simulink model "mavsim_chap6_week1"  (R2020b)
settings: Solver=ode4  StartTime=0.0  StopTime=tsim  FixedStep=P.Ts  RelTol=1e-3  EnableMultiTasking=on
InitFcn:
  | param_chap6
values from neighbouring files (symbols this model uses):
  aileron_c_sat = delta_a_max    (= 0.785398163397)    [runSim.m]
  closedLoopEnable = 1    [runSim.m]
  phi_c_sat = 45*pi/180    (= 0.785398163397)    [runSim.m]
undefined symbols (not defined in the file or in its folder): calc_chi, forces_moments, get_p, get_phi, P
libraries: simulink x3, pid_lib x2
settings Model: Creator=beard  LastModifiedBy=alanf
settings DataIOCC: LimitDataPoints=on  SaveFormat=Array  ReturnWorkspaceOutputs=off
settings OptimizationCC: ExpressionDepthLimit=2147483647  InitFltsAndDblsToZero=on  LifeSpan=inf
settings DebuggingCC: UnderspecifiedInitializationDetection=Classic  MergeDetectMultiDrivingBlocksExec=none  SolverPrmCheckMsg=warning  FcnCallInpInsideContextMsg=warning  StateNameClashWarn=warning  SFUnexpectedBacktrackingDiag=warning  SFNoUnconditionalDefaultTransitionDiag=warning  SFExecutionAtInitializationDiag=none  ArithmeticOperatorsInVariantConditions=warning
settings HardwareCC: ProdBitPerPointer=32  ProdBitPerSizeT=32  ProdBitPerPtrDiffT=32  ProdLargestAtomicFloat=None  ProdIntDivRoundTo=Undefined  ProdEndianess=Unspecified  ProdWordSize=32  ProdHWDeviceType=32-bit Generic
settings ModelReferenceCC: PropagateSignalLabelsOutOfModel=off
settings SFSimCC: SimUseLocalCustomCode=off  CustomCodeUndefinedFunction=UseInterfaceOnly
settings RTWCC: RTWUseLocalCustomCode=off
settings CodeAppCC: StateflowObjectComments=on
settings GRTTargetCC: TargetLangStandard=C89/C90 (ANSI)  CombineOutputUpdateFcns=off  GRTInterface=on
settings ConfigComp: CovMetricSettings=dw  CovSaveCumulativeToWorkspaceVar=on  CovSaveSingleToWorkspaceVar=on  CovExternalEMLEnable=off  CovSFcnEnable=off

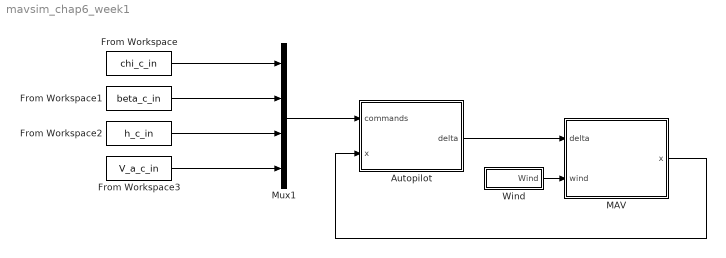
== system mavsim_chap6_week1 ==
  Autopilot : Subsystem
      mask Display: image(imread('kestrel.jpg'))
  From Workspace : FromWorkspace  VariableName=chi_c_in
  From Workspace1 : FromWorkspace  VariableName=beta_c_in
  From Workspace2 : FromWorkspace  VariableName=h_c_in
  From Workspace3 : FromWorkspace  VariableName=V_a_c_in
  MAV : Subsystem
      mask Display: image(imread('batcam.png'))
  Mux1 : Mux
  Wind : Subsystem
  wires:
  Wind/1(Wind) -> MAV/2(wind)
  MAV/1(x) -> Autopilot/2(x)
  Autopilot/1(delta) -> MAV/1(delta)
  Mux1/1 -> Autopilot/1(commands)
  From Workspace/1 -> Mux1/1
  From Workspace1/1 -> Mux1/2
  From Workspace2/1 -> Mux1/3
  From Workspace3/1 -> Mux1/4

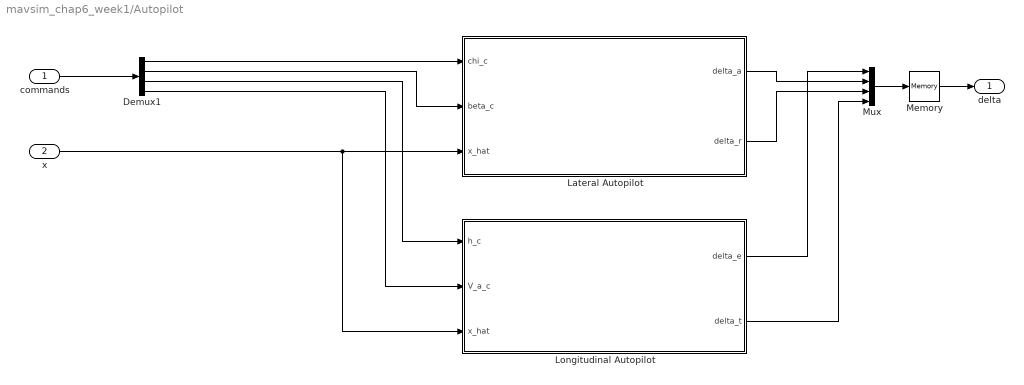
== system mavsim_chap6_week1/Autopilot ==
  commands : Inport
  x : Inport  Port=2
  Demux1 : Demux
  Lateral Autopilot : Subsystem
  Longitudinal Autopilot : Subsystem
  Memory : Memory  InitialCondition=P.u_trim  InheritSampleTime=on
  Mux : Mux
  delta : Outport  VectorParamsAs1DForOutWhenUnconnected=off
  wires:
  x/1 -> Longitudinal Autopilot/3(x_hat), Lateral Autopilot/3(x_hat)
  commands/1 -> Demux1/1
  Demux1/1 -> Lateral Autopilot/1(chi_c)
  Demux1/2 -> Lateral Autopilot/2(beta_c)
  Demux1/3 -> Longitudinal Autopilot/1(h_c)
  Demux1/4 -> Longitudinal Autopilot/2(V_a_c)
  Mux/1 -> Memory/1
  Memory/1 -> delta/1
  Longitudinal Autopilot/1(delta_e) -> Mux/1
  Lateral Autopilot/1(delta_a) -> Mux/2
  Lateral Autopilot/2(delta_r) -> Mux/3
  Longitudinal Autopilot/2(delta_t) -> Mux/4

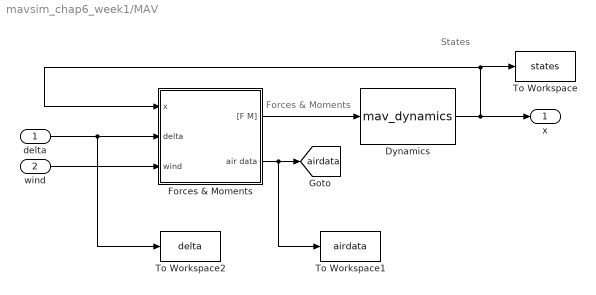
== system mavsim_chap6_week1/MAV ==
  note: Forces & Moments
  note: States
  delta : Inport
  wind : Inport  Port=2
  Dynamics : S-Function  FunctionName=mav_dynamics  Parameters=P  SFunctionDeploymentMode=off  EnableBusSupport=off
  Forces & Moments : Subsystem
  To Workspace : ToWorkspace  VariableName=states  SaveFormat=Timeseries  SampleTime=-1
  To Workspace1 : ToWorkspace  VariableName=airdata  SaveFormat=Timeseries  SampleTime=-1
  To Workspace2 : ToWorkspace  VariableName=delta  SaveFormat=Timeseries  SampleTime=-1
  x : Outport  VectorParamsAs1DForOutWhenUnconnected=off
  tag scope: airdata=global
  wires:
  Dynamics/1 -> Forces & Moments/1(x), To Workspace/1, x/1
  Forces & Moments/1("[F M]") -> Dynamics/1
  Forces & Moments/2(air data) -> To Workspace1/1, [airdata]
  delta/1 -> To Workspace2/1, Forces & Moments/2(delta)
  wind/1 -> Forces & Moments/3(wind)

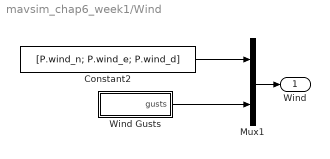
== system mavsim_chap6_week1/Wind ==
  Constant2 : Constant  Value=[P.wind_n; P.wind_e; P.wind_d]
  Mux1 : Mux  Inputs=2
  Wind Gusts : Subsystem
  Wind : Outport  VectorParamsAs1DForOutWhenUnconnected=off
  wires:
  Constant2/1 -> Mux1/1
  Mux1/1 -> Wind/1
  Wind Gusts/1(gusts) -> Mux1/2

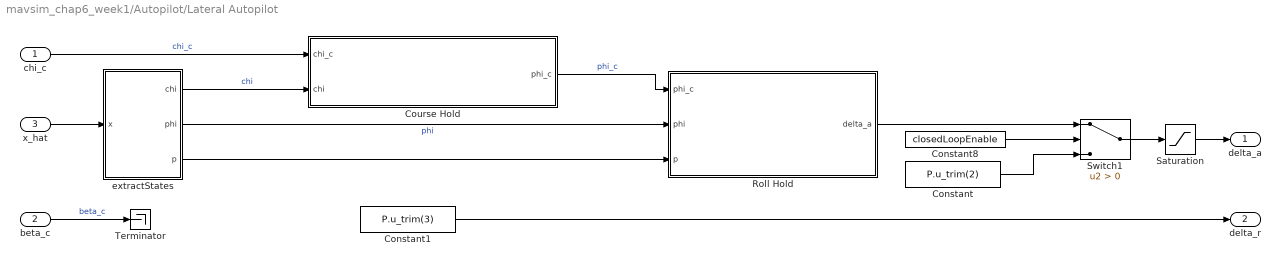
== system mavsim_chap6_week1/Autopilot/Lateral Autopilot ==
  chi_c : Inport
  beta_c : Inport  Port=2
  x_hat : Inport  Port=3
  Constant : Constant  Value=P.u_trim(2)
  Constant1 : Constant  Value=P.u_trim(3)
  Constant8 : Constant  Value=closedLoopEnable
  Course Hold : Subsystem
  Roll Hold : Subsystem
  Saturation : Saturate  UpperLimit=aileron_c_sat  LowerLimit=-aileron_c_sat
  Switch1 : Switch  Criteria=u2 > Threshold
  Terminator : Terminator
  extractStates : Subsystem
  delta_a : Outport  VectorParamsAs1DForOutWhenUnconnected=off
  delta_r : Outport  Port=2  VectorParamsAs1DForOutWhenUnconnected=off
  wires:
  chi_c/1 -> Course Hold/1(chi_c)  "chi_c"
  Course Hold/1(phi_c) -> Roll Hold/1(phi_c)  "phi_c"
  x_hat/1 -> extractStates/1(x)
  extractStates/1(chi) -> Course Hold/2(chi)  "chi"
  extractStates/2(phi) -> Roll Hold/2(phi)  "phi"
  extractStates/3(p) -> Roll Hold/3(p)
  Switch1/1 -> Saturation/1
  Constant/1 -> Switch1/3
  Roll Hold/1(delta_a) -> Switch1/1
  Constant8/1 -> Switch1/2
  Constant1/1 -> delta_r/1
  beta_c/1 -> Terminator/1  "beta_c"
  Saturation/1 -> delta_a/1

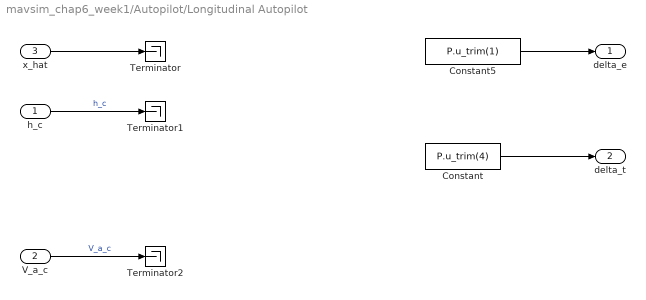
== system mavsim_chap6_week1/Autopilot/Longitudinal Autopilot ==
  h_c : Inport
  V_a_c : Inport  Port=2
  x_hat : Inport  Port=3
  Constant : Constant  Value=P.u_trim(4)
  Constant5 : Constant  Value=P.u_trim(1)
  Terminator : Terminator
  Terminator1 : Terminator
  Terminator2 : Terminator
  delta_e : Outport  VectorParamsAs1DForOutWhenUnconnected=off
  delta_t : Outport  Port=2  VectorParamsAs1DForOutWhenUnconnected=off
  wires:
  x_hat/1 -> Terminator/1
  h_c/1 -> Terminator1/1  "h_c"
  V_a_c/1 -> Terminator2/1  "V_a_c"
  Constant5/1 -> delta_e/1
  Constant/1 -> delta_t/1

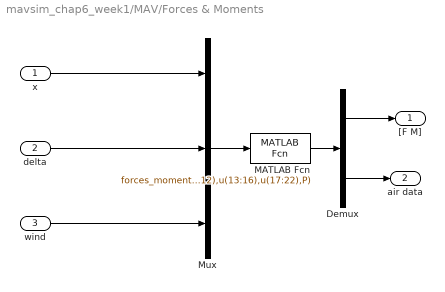
== system mavsim_chap6_week1/MAV/Forces & Moments ==
  x : Inport
  delta : Inport  Port=2
  wind : Inport  Port=3
  Demux : Demux  Outputs=[6;6]
  MATLAB Fcn : MATLABFcn  MATLABFcn=forces_moments(u(1:12),u(13:16),u(17:22),P)  OutputDimensions=12
  Mux : Mux  Inputs=3
  "[F M]" : Outport  VectorParamsAs1DForOutWhenUnconnected=off
  air data : Outport  Port=2  VectorParamsAs1DForOutWhenUnconnected=off
  wires:
  Demux/2 -> air data/1
  Mux/1 -> MATLAB Fcn/1
  Demux/1 -> "[F M]"/1
  MATLAB Fcn/1 -> Demux/1
  wind/1 -> Mux/3
  delta/1 -> Mux/2
  x/1 -> Mux/1

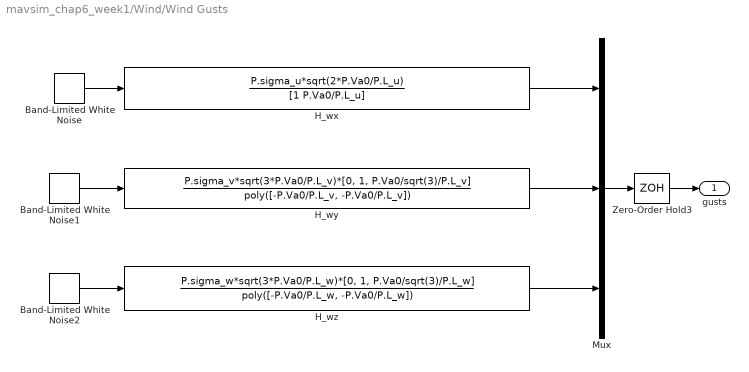
== system mavsim_chap6_week1/Wind/Wind Gusts ==
  Band-Limited White Noise : simulink/Sources/Band-Limited White Noise  Cov=[1]  Ts=P.Ts  seed=[23341]
  Band-Limited White Noise1 : simulink/Sources/Band-Limited White Noise  Cov=[1]  Ts=P.Ts  seed=[23341]
  Band-Limited White Noise2 : simulink/Sources/Band-Limited White Noise  Cov=[1]  Ts=P.Ts  seed=[23341]
  H_wx : TransferFcn  Numerator=P.sigma_u*sqrt(2*P.Va0/P.L_u)  Denominator=[1 P.Va0/P.L_u]
  H_wy : TransferFcn  Numerator=P.sigma_v*sqrt(3*P.Va0/P.L_v)*[0, 1, P.Va0/sqrt(3)/P.L_v]  Denominator=poly([-P.Va0/P.L_v, -P.Va0/P.L_v])
  H_wz : TransferFcn  Numerator=P.sigma_w*sqrt(3*P.Va0/P.L_w)*[0, 1, P.Va0/sqrt(3)/P.L_w]  Denominator=poly([-P.Va0/P.L_w, -P.Va0/P.L_w])
  Mux : Mux  Inputs=3
  Zero-Order Hold3 : ZeroOrderHold  SampleTime=P.Ts
  gusts : Outport  VectorParamsAs1DForOutWhenUnconnected=off
  wires:
  H_wx/1 -> Mux/1
  Band-Limited White Noise/1 -> H_wx/1
  H_wy/1 -> Mux/2
  Band-Limited White Noise1/1 -> H_wy/1
  H_wz/1 -> Mux/3
  Band-Limited White Noise2/1 -> H_wz/1
  Mux/1 -> Zero-Order Hold3/1
  Zero-Order Hold3/1 -> gusts/1

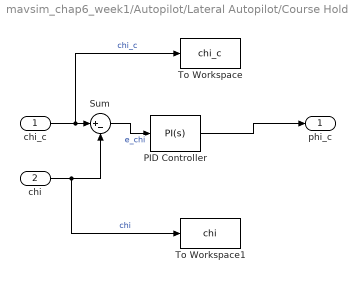
== system mavsim_chap6_week1/Autopilot/Lateral Autopilot/Course Hold ==
  chi_c : Inport
  chi : Inport  Port=2
  PID Controller : pid_lib/PID Controller  Controller=PI  Form=Parallel  TimeDomain=Continuous-time  UseExternalTs=off  SampleTime=-1  IntegratorMethod=Forward Euler  FilterMethod=Forward Euler  ControllerParametersSource=internal  P=P.k_pchi  I=P.k_ichi  D=0  UseFilter=on  N=100  TunerSelectOption=Transfer Function Based (PID Tuner App)  InitialConditionSource=internal  InitialConditionForIntegrator=0  InitialConditionForFilter=0  DifferentiatorICPrevScaledInput=0  ExternalReset=none  TrackingMode=off  Kt=1  LimitOutput=on  SatLimitsSource=internal  UpperSaturationLimit=phi_c_sat  LowerSaturationLimit=-phi_c_sat  LinearizeAsGain=on  AntiWindupMode=clamping  Kb=1  POutMin=[]  POutMax=[]  IOutMin=[]  IOutMax=[]  DOutMin=[]  DOutMax=[]  NOutMin=[]  NOutMax=[]  SumOutMin=[]  SumOutMax=[]  SaturationOutMin=[]  SaturationOutMax=[]  PParamMin=[]  PParamMax=[]  IParamMin=[]  IParamMax=[]  DParamMin=[]  DParamMax=[]  NParamMin=[]  NParamMax=[]  KbParamMin=[]  KbParamMax=[]  KtParamMin=[]  KtParamMax=[]  KbOutMin=[]  KbOutMax=[]  KtOutMin=[]  KtOutMax=[]  IntegratorOutMin=[]  IntegratorOutMax=[]  FilterOutMin=[]  FilterOutMax=[]  SumI1OutMin=[]  SumI1OutMax=[]  SumI2OutMin=[]  SumI2OutMax=[]  SumI3OutMin=[]  SumI3OutMax=[]  SumI4OutMin=[]  SumI4OutMax=[]  SumDOutMin=[]  SumDOutMax=[]  DifferentiatorOutMin=[]  DifferentiatorOutMax=[]  FilterDiffOutCoefMin=[]  FilterDiffOutCoefMax=[]  ReciprocalOutMin=[]  ReciprocalOutMax=[]  SumDenOutMin=[]  SumDenOutMax=[]  SumNumOutMin=[]  SumNumOutMax=[]  DivideOutMin=[]  DivideOutMax=[]  UdiffTsProdOutMin=[]  UdiffTsProdOutMax=[]  NTsProdOutMin=[]  NTsProdOutMax=[]  UintegralTsProdOutMin=[]  UintegralTsProdOutMax=[]  UngainTsProdOutMin=[]  UngainTsProdOutMax=[]  IntegratorContinuousStateAttributes=''  IntegratorStateMustResolveToSignalObject=off  IntegratorRTWStateStorageClass=Auto  FilterContinuousStateAttributes=''  FilterStateMustResolveToSignalObject=off  FilterRTWStateStorageClass=Auto  ParallelPVariant=InternalParameters  IdealPVariant=Disabled  IVariant=InternalParameters  DVariant=Disabled  IntegratorVariant=Continuous  SatVariant=Enabled  AWVariant=ContClampingParallel  PCopyVariant=Disabled  TRVariant=Disabled  FdbkBlocksVariant=Forward  IdealPFdbkVariant=Disabled  SatFdbkVariant=Disabled  DerivativeFilterVariant=Disabled  NVariant=Disabled  NCopyVariant=Disabled_SignalSpec  FilterICVariant=Disabled  IntegratorICVariant=InternalICs  ExternalResetVariant=Disabled  TRSumVariant=Passthrough  SumFdbkVariant=Disabled  SumVariant=Sum_PI  TsampFilterVariant=InternalTs  TsampNgainVariant=Passthrough  TsampIntegralVariant=Passthrough  ExternalSaturationOutDataTypeStr=Inherit: Same as second input
  Sum : Sum  Inputs=|+-
  To Workspace : ToWorkspace  VariableName=chi_c  SaveFormat=Timeseries  SampleTime=-1
  To Workspace1 : ToWorkspace  VariableName=chi  SaveFormat=Timeseries  SampleTime=-1
  phi_c : Outport  VectorParamsAs1DForOutWhenUnconnected=off
  wires:
  chi/1 -> Sum/2, To Workspace1/1  "chi"
  chi_c/1 -> Sum/1, To Workspace/1  "chi_c"
  Sum/1 -> PID Controller/1  "e_chi"
  PID Controller/1 -> phi_c/1

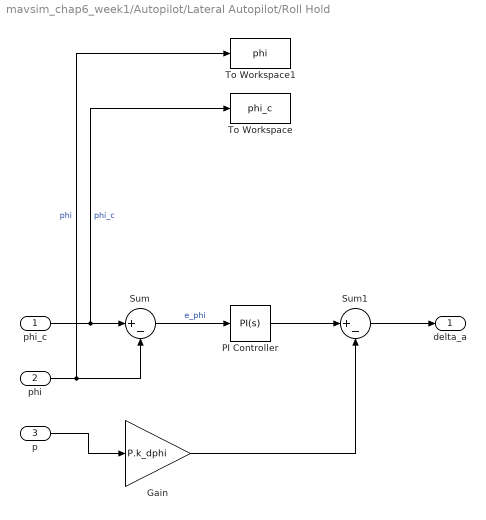
== system mavsim_chap6_week1/Autopilot/Lateral Autopilot/Roll Hold ==
  phi_c : Inport
  phi : Inport  Port=2
  p : Inport  Port=3
  Gain : Gain  Gain=P.k_dphi
  PI Controller : pid_lib/PID Controller  Controller=PI  Form=Parallel  TimeDomain=Continuous-time  UseExternalTs=off  SampleTime=-1  IntegratorMethod=Forward Euler  FilterMethod=Forward Euler  ControllerParametersSource=internal  P=P.k_pphi  I=P.k_iphi  D=0  UseFilter=on  N=100  TunerSelectOption=Transfer Function Based (PID Tuner App)  InitialConditionSource=internal  InitialConditionForIntegrator=0  InitialConditionForFilter=0  DifferentiatorICPrevScaledInput=0  ExternalReset=none  TrackingMode=off  Kt=1  LimitOutput=off  SatLimitsSource=internal  UpperSaturationLimit=inf  LowerSaturationLimit=-inf  LinearizeAsGain=on  AntiWindupMode=none  Kb=1  POutMin=[]  POutMax=[]  IOutMin=[]  IOutMax=[]  DOutMin=[]  DOutMax=[]  NOutMin=[]  NOutMax=[]  SumOutMin=[]  SumOutMax=[]  SaturationOutMin=[]  SaturationOutMax=[]  PParamMin=[]  PParamMax=[]  IParamMin=[]  IParamMax=[]  DParamMin=[]  DParamMax=[]  NParamMin=[]  NParamMax=[]  KbParamMin=[]  KbParamMax=[]  KtParamMin=[]  KtParamMax=[]  KbOutMin=[]  KbOutMax=[]  KtOutMin=[]  KtOutMax=[]  IntegratorOutMin=[]  IntegratorOutMax=[]  FilterOutMin=[]  FilterOutMax=[]  SumI1OutMin=[]  SumI1OutMax=[]  SumI2OutMin=[]  SumI2OutMax=[]  SumI3OutMin=[]  SumI3OutMax=[]  SumI4OutMin=[]  SumI4OutMax=[]  SumDOutMin=[]  SumDOutMax=[]  DifferentiatorOutMin=[]  DifferentiatorOutMax=[]  FilterDiffOutCoefMin=[]  FilterDiffOutCoefMax=[]  ReciprocalOutMin=[]  ReciprocalOutMax=[]  SumDenOutMin=[]  SumDenOutMax=[]  SumNumOutMin=[]  SumNumOutMax=[]  DivideOutMin=[]  DivideOutMax=[]  UdiffTsProdOutMin=[]  UdiffTsProdOutMax=[]  NTsProdOutMin=[]  NTsProdOutMax=[]  UintegralTsProdOutMin=[]  UintegralTsProdOutMax=[]  UngainTsProdOutMin=[]  UngainTsProdOutMax=[]  IntegratorContinuousStateAttributes=''  IntegratorStateMustResolveToSignalObject=off  IntegratorRTWStateStorageClass=Auto  FilterContinuousStateAttributes=''  FilterStateMustResolveToSignalObject=off  FilterRTWStateStorageClass=Auto  ParallelPVariant=InternalParameters  IdealPVariant=Disabled  IVariant=InternalParameters  DVariant=Disabled  IntegratorVariant=Continuous  SatVariant=Disabled  AWVariant=Passthrough  PCopyVariant=Disabled  TRVariant=Disabled  FdbkBlocksVariant=Forward  IdealPFdbkVariant=Disabled  SatFdbkVariant=Disabled  DerivativeFilterVariant=Disabled  NVariant=Disabled  NCopyVariant=Disabled_SignalSpec  FilterICVariant=Disabled  IntegratorICVariant=InternalICs  ExternalResetVariant=Disabled  TRSumVariant=Passthrough  SumFdbkVariant=Disabled  SumVariant=Sum_PI  TsampFilterVariant=InternalTs  TsampNgainVariant=Passthrough  TsampIntegralVariant=Passthrough  ExternalSaturationOutDataTypeStr=Inherit: Same as second input
  Sum : Sum  Inputs=|+-
  Sum1 : Sum  Inputs=|+-
  To Workspace : ToWorkspace  VariableName=phi_c  SaveFormat=Timeseries  SampleTime=-1
  To Workspace1 : ToWorkspace  VariableName=phi  SaveFormat=Timeseries  SampleTime=-1
  delta_a : Outport  VectorParamsAs1DForOutWhenUnconnected=off
  wires:
  phi_c/1 -> Sum/1, To Workspace/1  "phi_c"
  phi/1 -> To Workspace1/1, Sum/2  "phi"
  Sum/1 -> PI Controller/1  "e_phi"
  PI Controller/1 -> Sum1/1
  Sum1/1 -> delta_a/1
  p/1 -> Gain/1
  Gain/1 -> Sum1/2

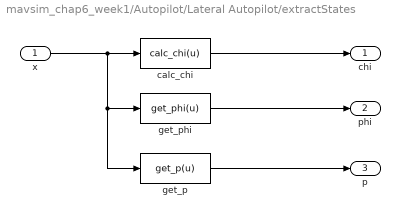
== system mavsim_chap6_week1/Autopilot/Lateral Autopilot/extractStates ==
  x : Inport
  calc_chi : MATLABFcn  MATLABFcn=calc_chi(u)
  get_p : MATLABFcn  MATLABFcn=get_p(u)
  get_phi : MATLABFcn  MATLABFcn=get_phi(u)
  chi : Outport  VectorParamsAs1DForOutWhenUnconnected=off
  phi : Outport  Port=2  VectorParamsAs1DForOutWhenUnconnected=off
  p : Outport  Port=3  VectorParamsAs1DForOutWhenUnconnected=off
  wires:
  x/1 -> get_p/1, get_phi/1, calc_chi/1
  calc_chi/1 -> chi/1
  get_phi/1 -> phi/1
  get_p/1 -> p/1
